simulink model "sus_4dof"  (R2019a)
settings: Solver=VariableStepAuto  StartTime=0.0  StopTime=10.0  RelTol=1e-3
settings Model: Creator=95865  LastModifiedBy=95865

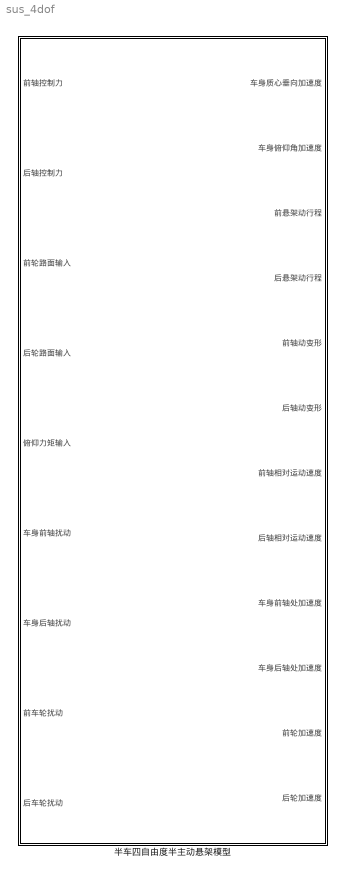
== system sus_4dof ==
  半车四自由度半主动悬架模型 : Subsystem  mask{mc=1, mtf=1, mtr=1, ksf=1, ksr=1, ktf=1, ktr=1, cof=1, cor=1, Ic=1, a=1, b=1, c_fmax=1}
      mask prompts: mc "簧载质量"; mtf "前悬架车轮质量"; mtr "后悬架车轮质量"; ksf "前悬架刚度"; ksr "后悬架刚度"; ktf "前轮胎刚度"; ktr "后轮胎刚度"; cof "前悬架磁流变阻尼器零场阻尼"; cor "后悬架磁流变阻尼器零场阻尼"; Ic "俯仰转动惯量"; a "质心到前轴距离"; b "质心到后轴距离"; c_fmax "磁流变阻尼器最大可调阻尼"

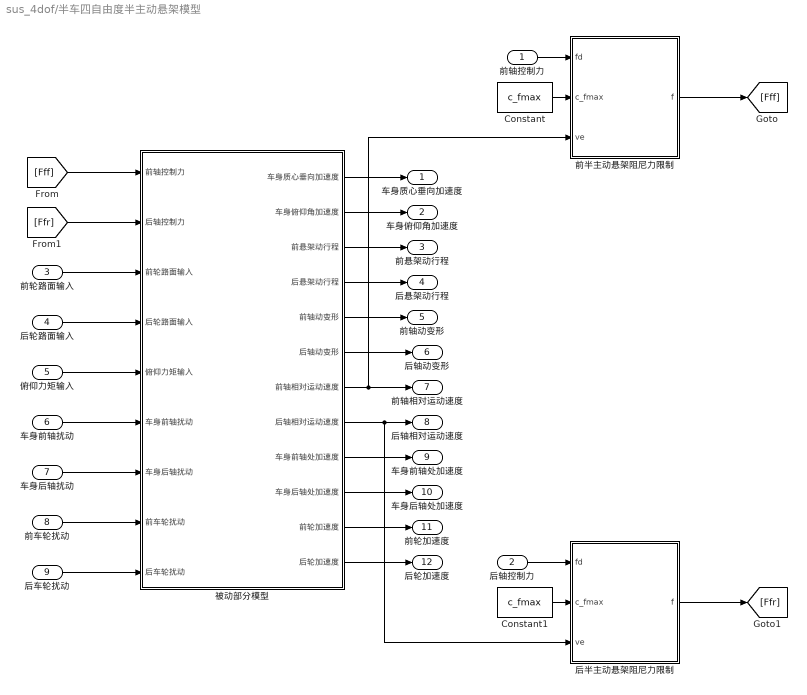
== system sus_4dof/半车四自由度半主动悬架模型 ==
  前轴控制力 : Inport
  后轴控制力 : Inport  Port=2
  前轮路面输入 : Inport  Port=3
  后轮路面输入 : Inport  Port=4
  俯仰力矩输入 : Inport  Port=5
  车身前轴扰动 : Inport  Port=6
  车身后轴扰动 : Inport  Port=7
  前车轮扰动 : Inport  Port=8
  后车轮扰动 : Inport  Port=9
  Constant : Constant  Value=c_fmax
  Constant1 : Constant  Value=c_fmax
  前半主动悬架阻尼力限制 : MATLAB Function  TreatAsAtomicUnit=on
  后半主动悬架阻尼力限制 : MATLAB Function  TreatAsAtomicUnit=on
  被动部分模型 : Subsystem
  车身质心垂向加速度 : Outport
  车身俯仰角加速度 : Outport  Port=2
  前悬架动行程 : Outport  Port=3
  后悬架动行程 : Outport  Port=4
  前轴动变形 : Outport  Port=5
  后轴动变形 : Outport  Port=6
  前轴相对运动速度 : Outport  Port=7
  后轴相对运动速度 : Outport  Port=8
  车身前轴处加速度 : Outport  Port=9
  车身后轴处加速度 : Outport  Port=10
  前轮加速度 : Outport  Port=11
  后轮加速度 : Outport  Port=12
  wires:
  前轮路面输入/1 -> 被动部分模型/3(前轮路面输入)
  后轮路面输入/1 -> 被动部分模型/4(后轮路面输入)
  俯仰力矩输入/1 -> 被动部分模型/5(俯仰力矩输入)
  车身前轴扰动/1 -> 被动部分模型/6(车身前轴扰动)
  车身后轴扰动/1 -> 被动部分模型/7(车身后轴扰动)
  前车轮扰动/1 -> 被动部分模型/8(前车轮扰动)
  后车轮扰动/1 -> 被动部分模型/9(后车轮扰动)
  被动部分模型/1(车身质心垂向加速度) -> 车身质心垂向加速度/1
  被动部分模型/2(车身俯仰角加速度) -> 车身俯仰角加速度/1
  被动部分模型/3(前悬架动行程) -> 前悬架动行程/1
  被动部分模型/4(后悬架动行程) -> 后悬架动行程/1
  被动部分模型/5(前轴动变形) -> 前轴动变形/1
  被动部分模型/6(后轴动变形) -> 后轴动变形/1
  被动部分模型/7(前轴相对运动速度) -> 前轴相对运动速度/1, 前半主动悬架阻尼力限制/3(ve)
  被动部分模型/8(后轴相对运动速度) -> 后轴相对运动速度/1, 后半主动悬架阻尼力限制/3(ve)
  Constant/1 -> 前半主动悬架阻尼力限制/2(c_fmax)
  前轴控制力/1 -> 前半主动悬架阻尼力限制/1(fd)
  [Fff] -> 被动部分模型/1(前轴控制力)
  后轴控制力/1 -> 后半主动悬架阻尼力限制/1(fd)
  Constant1/1 -> 后半主动悬架阻尼力限制/2(c_fmax)
  [Ffr] -> 被动部分模型/2(后轴控制力)
  前半主动悬架阻尼力限制/1(f) -> [Fff]
  后半主动悬架阻尼力限制/1(f) -> [Ffr]
  被动部分模型/9(车身前轴处加速度) -> 车身前轴处加速度/1
  被动部分模型/10(车身后轴处加速度) -> 车身后轴处加速度/1
  被动部分模型/11(前轮加速度) -> 前轮加速度/1
  被动部分模型/12(后轮加速度) -> 后轮加速度/1

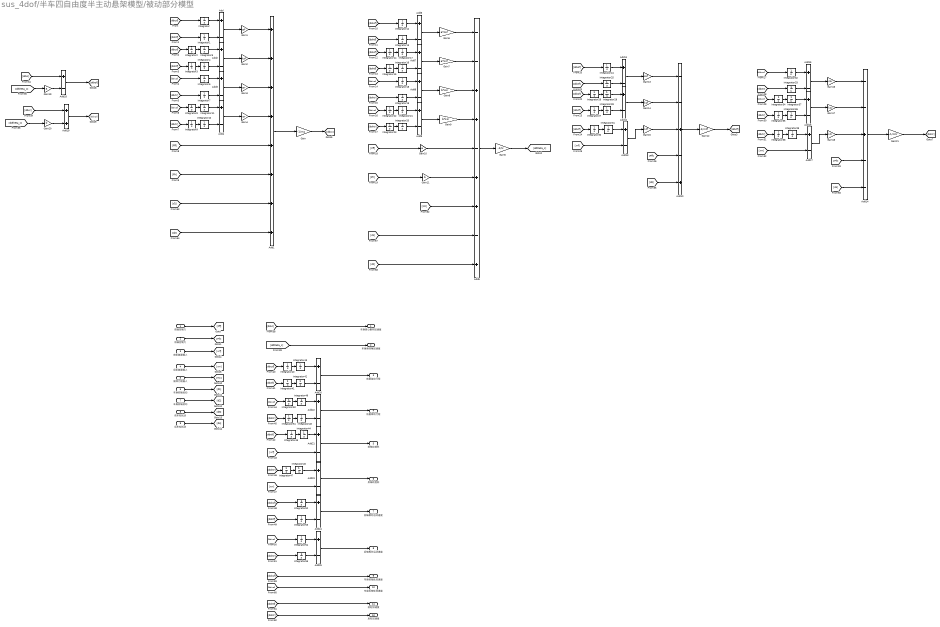
== system sus_4dof/半车四自由度半主动悬架模型/被动部分模型 ==
  前轴控制力 : Inport
  后轴控制力 : Inport  Port=2
  前轮路面输入 : Inport  Port=3
  后轮路面输入 : Inport  Port=4
  俯仰力矩输入 : Inport  Port=5
  车身前轴扰动 : Inport  Port=6
  车身后轴扰动 : Inport  Port=7
  前车轮扰动 : Inport  Port=8
  后车轮扰动 : Inport  Port=9
  Add{,2..4,6..9,11..13,15..18,20..25} (21 alike) : Sum  Inputs=+-
  Add1 : Sum  Inputs=++++++++
  Add10 : Sum  Inputs=--+-+
  Add14 : Sum  Inputs=--+--
  Add19 : Sum
  Add5 : Sum  Inputs=--++-++-+
  Gain : Gain  Gain=-1/mc
  Gain1 : Gain  Gain=cof
  Gain10 : Gain  Gain=a
  Gain11 : Gain  Gain=b
  Gain12 : Gain  Gain=-1/mtf
  Gain13 : Gain  Gain=cof
  Gain14 : Gain  Gain=ksf
  Gain15 : Gain  Gain=ktf
  Gain16 : Gain  Gain=cor
  Gain17 : Gain  Gain=ksr
  Gain18 : Gain  Gain=ktr
  Gain19 : Gain  Gain=a
  Gain2 : Gain  Gain=ksf
  Gain20 : Gain  Gain=b
  Gain21 : Gain  Gain=-1/mtr
  Gain3 : Gain  Gain=cor
  Gain4 : Gain  Gain=ksr
  Gain5 : Gain  Gain=-1/Ic
  Gain6 : Gain  Gain=a*cof
  Gain7 : Gain  Gain=a*ksf
  Gain8 : Gain  Gain=b*cor
  Gain9 : Gain  Gain=b*ksr
  Integrator{,1..55} (56 alike) : Integrator
  车身质心垂向加速度 : Outport
  车身俯仰角加速度 : Outport  Port=2
  前悬架动行程 : Outport  Port=3
  后悬架动行程 : Outport  Port=4
  前轴动变形 : Outport  Port=5
  后轴动变形 : Outport  Port=6
  前轴相对运动速度 : Outport  Port=7
  后轴相对运动速度 : Outport  Port=8
  车身前轴处加速度 : Outport  Port=9
  车身后轴处加速度 : Outport  Port=10
  前轮加速度 : Outport  Port=11
  后轮加速度 : Outport  Port=12
  wires:
  Add13/1 -> Gain15/1
  [ddxc] -> Add18/1
  [ddxsr] -> Integrator8/1
  Gain21/1 -> [ddxtr]
  [ddxsr] -> Integrator18/1
  [Fff] -> Gain10/1
  Integrator8/1 -> Integrator11/1
  Gain18/1 -> Add14/3
  Gain14/1 -> Add10/2
  [Fff] -> Add10/4
  Integrator26/1 -> Integrator29/1
  Integrator31/1 -> Add13/1
  车身前轴扰动/1 -> [d1]
  [d4] -> Add14/5
  [ddxtr] -> Integrator47/1
  [ddxtr] -> Integrator33/1
  [ddxtf] -> Integrator27/1
  [ddxsf] -> Integrator/1
  [xrr] -> Add17/2
  Add16/1 -> Gain17/1
  Add23/1 -> 后轴动变形/1
  Add17/1 -> Gain18/1
  Integrator1/1 -> Add/2
  Integrator43/1 -> Add20/1
  Gain13/1 -> Add10/1
  [ddxsf] -> Integrator26/1
  Gain7/1 -> Add5/2
  [ddxsf] -> Integrator52/1
  [xrf] -> Add21/2
  [d2] -> Add5/9
  [ddxsr] -> Integrator32/1
  Add8/1 -> Gain8/1
  [ddxsf] -> Integrator24/1
  Add18/1 -> [ddxsf]
  Integrator6/1 -> Add3/1
  Integrator21/1 -> Add9/1
  Integrator27/1 -> Integrator28/1
  Integrator16/1 -> Add7/2
  Gain5/1 -> [ddtheta_c]
  Integrator40/1 -> Integrator43/1
  Add15/1 -> Gain16/1
  Gain4/1 -> Add1/4
  Integrator34/1 -> Integrator37/1
  Add7/1 -> Gain7/1
  [ddxtr] -> Integrator35/1
  Gain20/1 -> Add19/2
  Integrator36/1 -> Add16/2
  Integrator53/1 -> Add24/2
  [xrf] -> Add13/2
  [ddxtr] -> Integrator51/1
  [ddtheta_c] -> Gain19/1
  Gain17/1 -> Add14/2
  Gain1/1 -> Add1/1
  Integrator35/1 -> Integrator36/1
  [ddxsf] -> Integrator14/1
  Gain/1 -> [ddxc]
  Gain6/1 -> Add5/1
  Add2/1 -> Gain2/1
  Integrator37/1 -> Add16/1
  Integrator28/1 -> Add12/2
  [ddxtr] -> Integrator38/1
  [ddxtr] -> Integrator9/1
  [ddxtr] -> Integrator23/1
  Add19/1 -> [ddxsr]
  [ddxsr] -> Integrator50/1
  Integrator15/1 -> Integrator16/1
  Integrator32/1 -> Add15/1
  Integrator48/1 -> Add22/2
  [ddxtf] -> Integrator1/1
  Integrator5/1 -> Add2/1
  [xrr] -> Add23/2
  Integrator22/1 -> Integrator21/1
  Integrator10/1 -> Add4/2
  [ddxc] -> Add19/1
  Integrator4/1 -> Add2/2
  [ddxsf] -> Integrator40/1
  Gain15/1 -> Add10/3
  [ddxtf] -> Integrator41/1
  Gain8/1 -> Add5/3
  Add20/1 -> 前悬架动行程/1
  [ddtheta_c] -> Gain20/1
  Gain19/1 -> Add18/2
  Integrator41/1 -> Integrator42/1
  Add22/1 -> 后悬架动行程/1
  Integrator45/1 -> Integrator44/1
  Gain2/1 -> Add1/2
  Add5/1 -> Gain5/1
  Add21/1 -> 前轴动变形/1
  Integrator38/1 -> Integrator39/1
  Integrator52/1 -> Add24/1
  [ddxtf] -> Integrator25/1
  Add/1 -> Gain1/1
  Integrator51/1 -> Integrator48/1
  Integrator24/1 -> Add11/1
  [ddxtf] -> Integrator45/1
  Integrator55/1 -> Add25/2
  [ddxtr] -> Integrator55/1
  [ddxtf] -> Integrator53/1
  Integrator54/1 -> Add25/1
  Add24/1 -> 前轴相对运动速度/1
  Integrator19/1 -> Add8/2
  [ddxsf] -> Integrator2/1
  Integrator7/1 -> Add3/2
  [ddxtf] -> Integrator30/1
  [ddxsr] -> Integrator54/1
  Add25/1 -> 后轴相对运动速度/1
  Add12/1 -> Gain14/1
  Integrator33/1 -> Add15/2
  Gain11/1 -> Add5/6
  [Mc] -> Add5/7
  Integrator49/1 -> Add22/1
  [d1] -> Add1/7
  Integrator47/1 -> Integrator46/1
  Integrator13/1 -> Add6/2
  Integrator42/1 -> Add20/2
  [d1] -> Add5/8
  Integrator46/1 -> Add23/1
  [d2] -> Add1/8
  [ddxsr] -> Integrator22/1
  [ddxsr] -> Integrator34/1
  [d3] -> Add10/5
  Integrator50/1 -> Integrator49/1
  Integrator30/1 -> Integrator31/1
  Integrator29/1 -> Add12/1
  Integrator20/1 -> Add9/2
  Integrator44/1 -> Add21/1
  Add9/1 -> Gain9/1
  Integrator39/1 -> Add17/1
  Add4/1 -> Gain4/1
  Gain3/1 -> Add1/3
  Integrator17/1 -> Add7/1
  Integrator/1 -> Add/1
  Integrator3/1 -> Integrator4/1
  Integrator2/1 -> Integrator5/1
  Integrator11/1 -> Add4/1
  [ddxtf] -> Integrator3/1
  [ddxsr] -> Integrator6/1
  Integrator9/1 -> Integrator10/1
  Add3/1 -> Gain3/1
  Add6/1 -> Gain6/1
  [Ffr] -> Add1/6
  Integrator12/1 -> Add6/1
  [Fff] -> Add1/5
  [ddxtr] -> Integrator7/1
  [ddxsf] -> Integrator12/1
  [ddxtf] -> Integrator15/1
  [ddxtf] -> Integrator13/1
  [ddxtr] -> Integrator19/1
  Add11/1 -> Gain13/1
  Integrator18/1 -> Add8/1
  [Ffr] -> Gain11/1
  Integrator23/1 -> Integrator20/1
  Integrator25/1 -> Add11/2
  Integrator14/1 -> Integrator17/1
  Gain9/1 -> Add5/4
  Gain10/1 -> Add5/5
  Add10/1 -> Gain12/1
  后车轮扰动/1 -> [d4]
  [Ffr] -> Add14/4
  Gain16/1 -> Add14/1
  俯仰力矩输入/1 -> [Mc]
  [ddtheta_c] -> 车身俯仰角加速度/1
  后轮路面输入/1 -> [xrr]
  [ddxc] -> 车身质心垂向加速度/1
  车身后轴扰动/1 -> [d2]
  前车轮扰动/1 -> [d3]
  前轴控制力/1 -> [Fff]
  Add1/1 -> Gain/1
  Gain12/1 -> [ddxtf]
  后轴控制力/1 -> [Ffr]
  前轮路面输入/1 -> [xrf]
  Add14/1 -> Gain21/1
  [ddxsf] -> 车身前轴处加速度/1
  [ddxsr] -> 车身后轴处加速度/1
  [ddxtf] -> 前轮加速度/1
  [ddxtr] -> 后轮加速度/1

== matlab function sus_4dof/半车四自由度半主动悬架模型/后半主动悬架阻尼力限制 ==
  data: fd input; f output; c_fmax input; ve input
function f  = fcn(fd, c_fmax,ve)
if fd/ve>c_fmax
    f=c_fmax*ve;
elseif (fd/ve<=c_fmax)&&(fd/ve>0)
    f=fd;
else
    f=0;
end 

end

== matlab function sus_4dof/半车四自由度半主动悬架模型/前半主动悬架阻尼力限制 ==
  data: fd input; f output; c_fmax input; ve input
function f  = fcn(fd, c_fmax,ve)
if fd/ve>c_fmax
    f=c_fmax*ve;
elseif (fd/ve<=c_fmax)&&(fd/ve>0)
    f=fd;
else
    f=0;
end 

end
